simulink library "pingcap"  (R2021a)
settings: Solver=VariableStepAuto  StartTime=0.0  StopTime=10.0  RelTol=1e-3
libraries: $bdroot x5
settings Model: Creator=tongjian  LastModifiedBy=tongjian

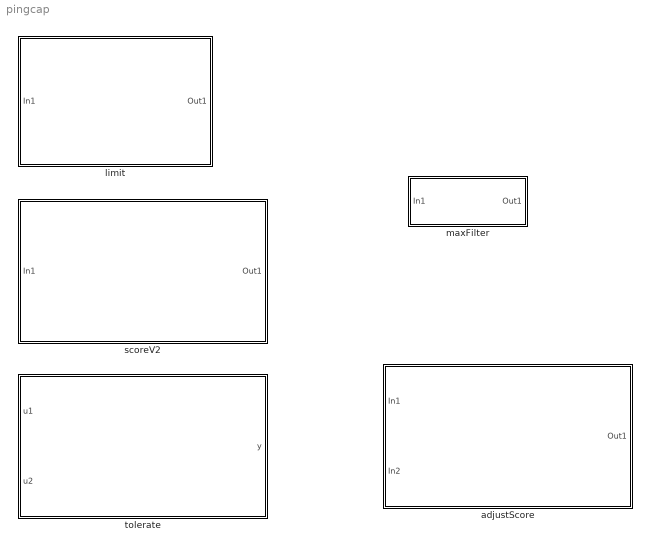
== system pingcap ==
  adjustScore : Subsystem
  limit : Subsystem  mask(limit){g_limit=0, g_value=0}
      mask prompts: g_limit "limit"; g_value "value"
      mask help:
      | limit if x>limt y=v
      | elseif x<-limit y=-v
      | else 0
      mask Display: disp('limit if x>limt y=v elseif x<-limit y=-v  ')
  maxFilter : Subsystem  mask{g_n=0, g_Ts=0}
      mask prompts: g_n "n"; g_Ts "Ts"
  scoreV2 : Subsystem  mask{g_lowSpaceRatio=0, g_amp=0, g_capacity=0}
      mask prompts: g_lowSpaceRatio "lowSpaceRatio"; g_amp "amp"; g_capacity "capacity"
      mask Display: disp('scoreV2')
  tolerate : Subsystem  mask{g_tolerateSize=0}
      mask prompts: g_tolerateSize "tolerateSize"
      mask Display: disp('tolerate')

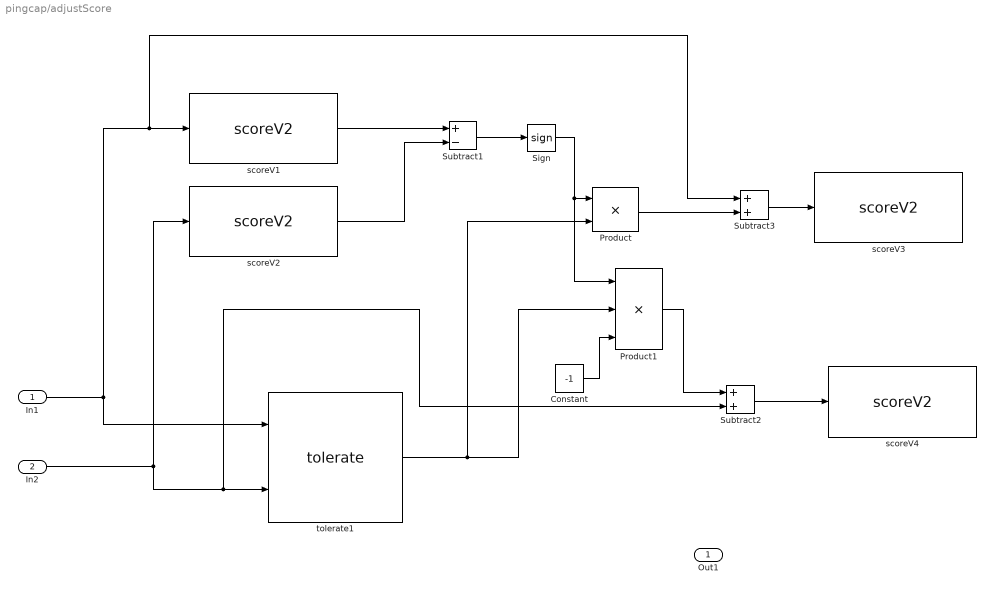
== system pingcap/adjustScore ==
  In1 : Inport
  In2 : Inport  Port=2
  Constant : Constant  Value=-1
  Product : Product
  Product1 : Product  Inputs=3
  Sign : Signum
  Subtract1 : Sum  Inputs=+-
  Subtract2 : Sum
  Subtract3 : Sum
  scoreV{1..4} (4 alike) : $bdroot/scoreV2  g_lowSpaceRatio=0  g_amp=0  g_capacity=0
  tolerate1 : $bdroot/tolerate  g_tolerateSize=0
  Out1 : Outport
  wires:
  In2/1 -> scoreV2/1, Subtract2/2, tolerate1/2
  In1/1 -> Subtract3/1, scoreV1/1, tolerate1/1
  scoreV1/1 -> Subtract1/1
  scoreV2/1 -> Subtract1/2
  tolerate1/1 -> Product/2, Product1/2
  Product1/1 -> Subtract2/1
  Subtract3/1 -> scoreV3/1
  Subtract1/1 -> Sign/1
  Sign/1 -> Product1/1, Product/1
  Constant/1 -> Product1/3
  Product/1 -> Subtract3/2
  Subtract2/1 -> scoreV4/1

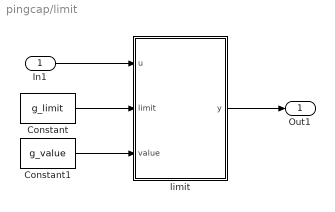
== system pingcap/limit ==
  In1 : Inport
  Constant : Constant  Value=g_limit
  Constant1 : Constant  Value=g_value
  limit : MATLAB Function  TreatAsAtomicUnit=on
  Out1 : Outport
  wires:
  In1/1 -> limit/1(u)
  limit/1(y) -> Out1/1
  Constant/1 -> limit/2(limit)
  Constant1/1 -> limit/3(value)

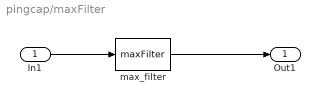
== system pingcap/maxFilter ==
  In1 : Inport
  max_filter : M-S-Function  FunctionName=maxFilter  Parameters=(g_n,g_Ts)
  Out1 : Outport
  wires:
  In1/1 -> max_filter/1
  max_filter/1 -> Out1/1

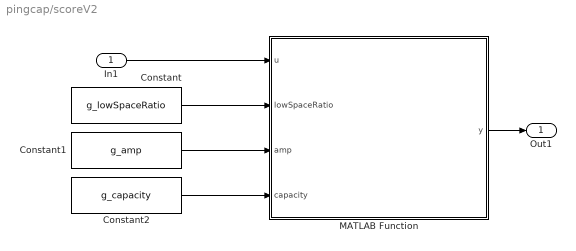
== system pingcap/scoreV2 ==
  In1 : Inport
  Constant : Constant  Value=g_lowSpaceRatio
  Constant1 : Constant  Value=g_amp
  Constant2 : Constant  Value=g_capacity
  MATLAB Function : MATLAB Function  TreatAsAtomicUnit=on
  Out1 : Outport
  wires:
  In1/1 -> MATLAB Function/1(u)
  MATLAB Function/1(y) -> Out1/1
  Constant/1 -> MATLAB Function/2(lowSpaceRatio)
  Constant1/1 -> MATLAB Function/3(amp)
  Constant2/1 -> MATLAB Function/4(capacity)

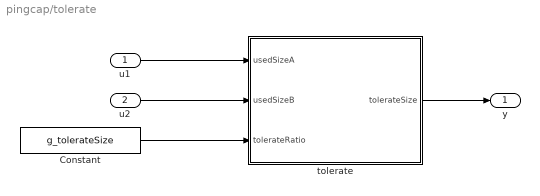
== system pingcap/tolerate ==
  u1 : Inport
  u2 : Inport  Port=2
  Constant : Constant  Value=g_tolerateSize
  tolerate : MATLAB Function  TreatAsAtomicUnit=on
  y : Outport
  wires:
  u1/1 -> tolerate/1(usedSizeA)
  u2/1 -> tolerate/2(usedSizeB)
  Constant/1 -> tolerate/3(tolerateRatio)
  tolerate/1(tolerateSize) -> y/1

== matlab function pingcap/scoreV2/MATLAB Function ==
  data: u input; y output; lowSpaceRatio input; amp input; capacity input
% u: used size ,unit:Gb
% capacity: disk space 
function y = fcn(u,lowSpaceRatio,amp,capacity)
k=1;
m=256;
b=1e7;
f=50; 
if f<capacity*(1-lowSpaceRatio)
    f=capacity*(1-lowSpaceRatio);
end
%  available 
a=capacity-u;
r=u*amp*1024;

if a>f
    b=a-f+1;
    y=(k*r+m*(log(capacity)-log(b))/(capacity-b)*r);
else
    y=(k+m*log(capacity)/capacity)*r+b*(f-a)/f;
end

== matlab function pingcap/limit/limit ==
  data: u input; y output; limit input; value input
function y = fcn(u,limit,value)
if u>limit 
    y=value;
elseif u<-limit
    y=-value;
else
    y=0;
end

== matlab function pingcap/tolerate/tolerate ==
  data: usedSizeA input; tolerateSize output; usedSizeB input; tolerateRatio input
function tolerateSize = fcn(usedSizeA, usedSizeB, tolerateRatio)
% regionSize=96MB
regionSize=96;
minTolerantSizeRatio=1.0;
adjustRatio=0.005;

size=max(usedSizeA,usedSizeB);
tolerateCount=tolerateRatio;
if tolerateRatio==0
    tolerateCount=max(minTolerantSizeRatio,size*1024/regionSize*adjustRatio);
end

tolerateSize=regionSize*tolerateCount/1024;
